simulink model "nco_lut_direct"  (R2016a)
settings: Solver=VariableStepAuto  StartTime=0.0  StopTime=10.0  RelTol=1e-3
libraries: simulink x3
settings Model: Creator=sj660  LastModifiedBy=sj660

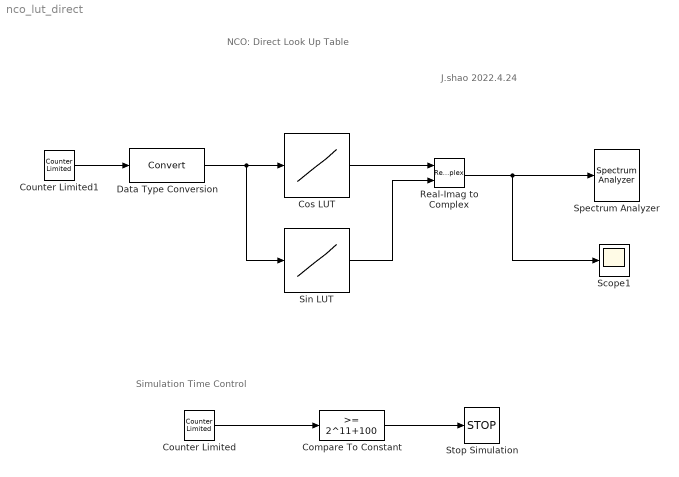
== system nco_lut_direct ==
  note: Simulation Time Control
  note: NCO: Direct Look Up Table
  note: J.shao 2022.4.24
  Compare To Constant : simulink/Logic and Bit Operations/Compare To Constant  relop=>=  const=2^11+100  OutDataTypeStr=boolean
  Cos LUT : Lookup_n-D  NumberOfTableDimensions=1  BreakpointsForDimension1=[0:1:1023]  BreakpointsForDimension1FirstPoint=0  UseOneInputPortForAllInputData=on  Table=cos([0:2*pi/1024:2*pi-2*pi/1024])  InterpMethod=Nearest  ExtrapMethod=Cubic spline  InternalRulePriority=Speed  OutDataTypeStr=fixdt(1,13,11)  RndMeth=Simplest  InputSameDT=on
  Counter Limited : simulink/Sources/Counter Limited  uplimit=2^12  tsamp=1e-9
  Counter Limited1 : simulink/Sources/Counter Limited  uplimit=2^10-1  tsamp=1e-9
  Data Type Conversion : DataTypeConversion
  Real-Imag to Complex : RealImagToComplex
  Scope1 : Scope
  Sin LUT : Lookup_n-D  NumberOfTableDimensions=1  BreakpointsForDimension1=[0:1:1023]  BreakpointsForDimension1FirstPoint=0  UseOneInputPortForAllInputData=on  Table=sin([0:2*pi/1024:2*pi-2*pi/1024])  InterpMethod=Nearest  ExtrapMethod=Cubic spline  InternalRulePriority=Speed  OutDataTypeStr=fixdt(1,13,11)  RndMeth=Simplest  InputSameDT=on
  Spectrum Analyzer : SpectrumAnalyzer
  Stop Simulation : Stop
  wires:
  Counter Limited/1 -> Compare To Constant/1
  Compare To Constant/1 -> Stop Simulation/1
  Counter Limited1/1 -> Data Type Conversion/1
  Data Type Conversion/1 -> Sin LUT/1, Cos LUT/1
  Real-Imag to Complex/1 -> Spectrum Analyzer/1, Scope1/1
  Cos LUT/1 -> Real-Imag to Complex/1
  Sin LUT/1 -> Real-Imag to Complex/2
